simulink model "SimulacionMotorDCsimulink"  (R2017b)
settings: Solver=VariableStepAuto  StartTime=0.0  StopTime=6  RelTol=1e-3
values from neighbouring files (symbols this model uses):
  A = [-b/J   K/J ... (first row only)    [SimuladoMotorDC.m]
  B = [0 ... (first row only)    [SimuladoMotorDC.m]
  C = [1   0]    [SimuladoMotorDC.m]
  D = 0    [SimuladoMotorDC.m]
  dem = [L*J R*J+b*L K^2+b*R]    [SimuladoMotorDC.m]
  num = K    (= 0.01)    [SimuladoMotorDC.m]
settings Model: Creator=Leonardo  LastModifiedBy=Leonardo

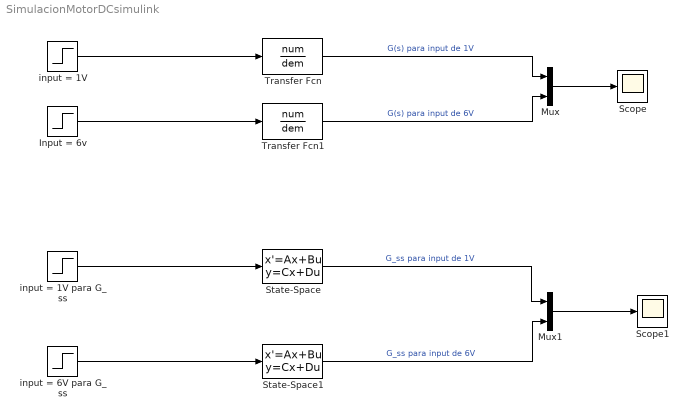
== system SimulacionMotorDCsimulink ==
  Input = 6v : Step  Time=2  After=6  SampleTime=0
  Mux : Mux  Inputs=2
  Mux1 : Mux  Inputs=2
  Scope : Scope
  Scope1 : Scope
  State-Space : StateSpace  A=A  B=B  C=C  D=D  InitialCondition=0
  State-Space1 : StateSpace  A=A  B=B  C=C  D=D  InitialCondition=0
  Transfer Fcn : TransferFcn  Numerator=num  Denominator=dem
  Transfer Fcn1 : TransferFcn  Numerator=num  Denominator=dem
  input = 1V : Step  Time=2  SampleTime=0
  input = 1V para G_ss : Step  Time=2  SampleTime=0
  input = 6V para G_ss : Step  Time=2  After=6  SampleTime=0
  wires:
  input = 1V/1 -> Transfer Fcn/1
  Mux/1 -> Scope/1
  Input = 6v/1 -> Transfer Fcn1/1
  Transfer Fcn/1 -> Mux/1  "G(s) para input de 1V"
  Transfer Fcn1/1 -> Mux/2  "G(s) para input de 6V"
  input = 1V para G_ss/1 -> State-Space/1
  Mux1/1 -> Scope1/1
  input = 6V para G_ss/1 -> State-Space1/1
  State-Space/1 -> Mux1/1  "G_ss para input de 1V"
  State-Space1/1 -> Mux1/2  "G_ss para input de 6V"
